simulink model "GaNModel_Nonsegmented"  (R2016a)
settings: Solver=VariableStepAuto  StartTime=0.0  StopTime=4e-5  MaxStep=0.01  RelTol=1e-3
values from neighbouring files (symbols this model uses):
  b1 = -8.43    [CapacitanceAnalytical.m]    (also in GanModel_Nonsegmented.m = 2.035; HalfBridge.m = 2.035; PoleZero.m = 3.944609415e-18)
  b2 = 42.2    [CapacitanceAnalytical.m]    (also in GanModel_Nonsegmented.m = 2.054; HalfBridge.m = 2.054; PoleZero.m = 7.00901047e-28)
  c1 = 30.26    [CapacitanceAnalytical.m]    (also in GanModel_Nonsegmented.m = 0.124; HalfBridge.m = 0.124; PoleZero.m = 5.00726198929e-08)
  c2 = 7.341    [CapacitanceAnalytical.m]    (also in GanModel_Nonsegmented.m = 0.153; HalfBridge.m = 0.153; PoleZero.m = 1.94274928479e-17)
  Cds = Coss - Crss    [CapacitanceAnalytical.m]    (also in GanModel_Nonsegmented.m = 1.65e-11; HalfBridge.m = 6.3e-11; HalfBridgeBottomConnectedLoad.m = 6.3e-11; HalfBridgeCapacitanceModelling.m = 6.3e-11)
  Cgd = Crss    [CapacitanceAnalytical.m]    (also in GanModel_Nonsegmented.m = 5e-13; HalfBridge.m = 2e-12; HalfBridgeBottomConnectedLoad.m = 2e-12; HalfBridgeCapacitanceModelling.m = 2e-12)
  Cgs = Ciss - Crss    [CapacitanceAnalytical.m]    (also in GanModel_Nonsegmented.m = 6.45e-11; HalfBridge.m = 2.58e-10; HalfBridgeBottomConnectedLoad.m = 2.58e-10; HalfBridgeCapacitanceModelling.m = 2.58e-10)
  d1 = 1.159    [GanModel_Nonsegmented.m]    (also in HalfBridge.m)
  e1 = -0.204    [GanModel_Nonsegmented.m]    (also in HalfBridge.m)
  fsw = 1e6    (= 1000000)    [ChannelAndDSTrajectories.m]    (also in GanModel_Nonsegmented.m = 100000; HalfBridge.m; HalfBridgeBottomConnectedLoad.m; HalfBridgeCapacitanceModelling.m)
  K1 = 0.283    [GanModel_Nonsegmented.m]    (also in HalfBridge.m)
  K2 = 7.114    [GanModel_Nonsegmented.m]    (also in HalfBridge.m)
  Ld = 10e-9    (= 1e-08)    [GanModel_Nonsegmented.m]    (also in HalfBridge.m = 7e-09; HalfBridgeBottomConnectedLoad.m = 7e-09; HalfBridgeCapacitanceModelling.m = 7e-10)
  m1 = 30.972    [GanModel_Nonsegmented.m]    (also in HalfBridge.m)
  n1 = -4.48    [GanModel_Nonsegmented.m]    (also in HalfBridge.m)
  PulseAmplitude = 5    [GanModel_Nonsegmented.m]    (also in HalfBridge.m; HalfBridgeBottomConnectedLoad.m; HalfBridgeCapacitanceModelling.m)
  Rd = 3.6*0.95*0.82*18.2*0.25/295    (= 0.0432543050847)    [AnalyticalModel.m]    (also in GanModel_Nonsegmented.m = 0.1; HalfBridge.m = 2.5e-05; HalfBridgeBottomConnectedLoad.m = 2.5e-05; HalfBridgeCapacitanceModelling.m = 2.5e-05)
  Rg = 1    [GanModel_Nonsegmented.m]    (also in HalfBridge.m; HalfBridgeBottomConnectedLoad.m = 1.5; HalfBridgeCapacitanceModelling.m = 1.5)
  Rs = 3.6*0.238*0.82/295    (= 0.00238161355932)    [AnalyticalModel.m]    (also in GanModel_Nonsegmented.m = 0.1; HalfBridge.m = 2.5e-05; HalfBridgeBottomConnectedLoad.m = 2.5e-05; HalfBridgeCapacitanceModelling.m = 2.5e-05)
  SampleTime = 1e-12    [GanModel_Nonsegmented.m]    (also in HalfBridge.m = 5e-13; HalfBridgeBottomConnectedLoad.m = 5e-13; HalfBridgeCapacitanceModelling.m = 5e-13)
  Vdc = 300    [GanModel_Nonsegmented.m]    (also in HalfBridge.m; HalfBridgeBottomConnectedLoad.m; HalfBridgeCapacitanceModelling.m)
libraries: powerlib x18
settings Model: Creator=ugurm  LastModifiedBy=ugurm
settings DebuggingCC: UnconnectedInputMsg=none  UnconnectedOutputMsg=none  UnconnectedLineMsg=none

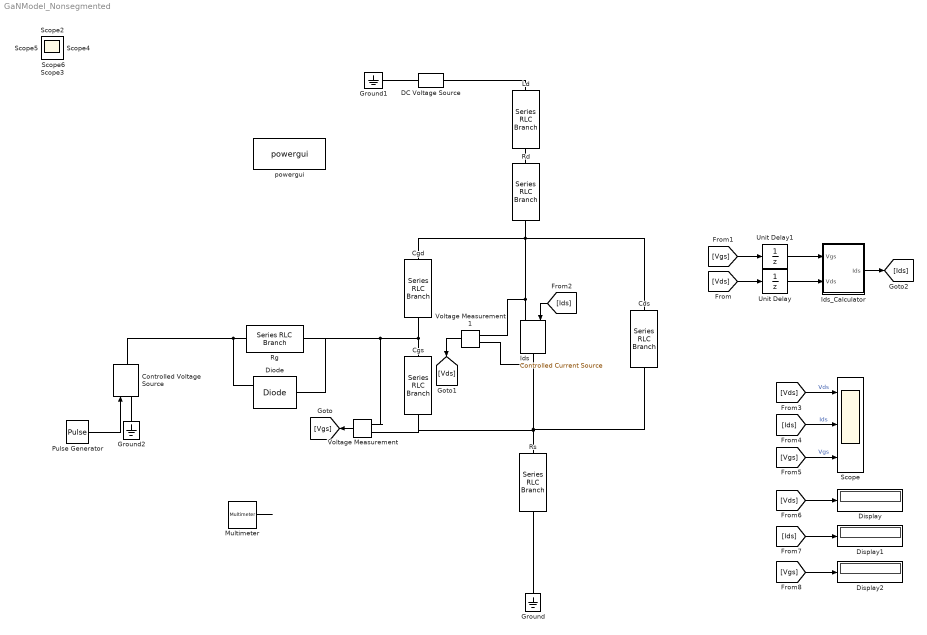
== system GaNModel_Nonsegmented ==
  Cds : powerlib/Elements/Series RLC Branch  LConnTagsString=__new0  RConnTagsString=__new0  BranchType=C  Resistance=1  Inductance=1e-3  SetiL0=off  InitialCurrent=0  Capacitance=Cds  Setx0=off  InitialVoltage=0  Measurements=None
  Cgd : powerlib/Elements/Series RLC Branch  LConnTagsString=__new0  RConnTagsString=__new0  BranchType=C  Resistance=1  Inductance=1e-3  SetiL0=off  InitialCurrent=0  Capacitance=Cgd  Setx0=off  InitialVoltage=0  Measurements=None
  Cgs : powerlib/Elements/Series RLC Branch  LConnTagsString=__new0  RConnTagsString=__new0  BranchType=C  Resistance=1  Inductance=1e-3  SetiL0=off  InitialCurrent=0  Capacitance=Cgs  Setx0=off  InitialVoltage=0  Measurements=None
  Controlled Voltage Source : powerlib/Electrical Sources/Controlled Voltage Source  Initialize=off  Source_Type=AC  Amplitude=0  Phase=0  Frequency=0  Measurements=Voltage
  DC Voltage Source : powerlib/Electrical Sources/DC Voltage Source  Amplitude=Vdc  Measurements=None
  Diode : powerlib/Power Electronics/Diode  Ron=0.001  Lon=0  Vf=0.8  IC=0  UseSnubber=off  Rs=500  Cs=250e-9  Measurements=on
  Display : Display
  Display1 : Display
  Display2 : Display
  Ground : powerlib/Elements/Ground  LConnTagsString=a
  Ground1 : powerlib/Elements/Ground  LConnTagsString=a
  Ground2 : powerlib/Elements/Ground  LConnTagsString=a
  Ids : powerlib/Electrical Sources/Controlled Current Source  Initialize=on  Source_Type=AC  Amplitude=0  Phase=0  Frequency=0  Measurements=None
  Ids_Calculator : Subsystem
  Ld : powerlib/Elements/Series RLC Branch  LConnTagsString=__new0  RConnTagsString=__new0  BranchType=L  Resistance=Rd  Inductance=Ld  SetiL0=off  InitialCurrent=0  Capacitance=1e-6  Setx0=off  InitialVoltage=0  Measurements=None
  Multimeter : powerlib/Measurements/Multimeter  PhasorSimulation=off  OutputType=Complex  sel=1  L=1  Gain=1  yselected={'Usrc: Controlled Voltage Source'};  PSBOutputType=1  PSBequivalent=0  AxesSetting=[0,0.1,-100,100]  Display=0  SavedBlockNames=-11
  Pulse Generator : DiscretePulseGenerator  PulseType=Time based  Amplitude=PulseAmplitude  Period=1/fsw  PulseWidth=50
  Rd : powerlib/Elements/Series RLC Branch  LConnTagsString=__new0  RConnTagsString=__new0  BranchType=R  Resistance=Rd  Inductance=1e-3  SetiL0=off  InitialCurrent=0  Capacitance=1e-6  Setx0=off  InitialVoltage=0  Measurements=None
  Rg : powerlib/Elements/Series RLC Branch  LConnTagsString=__new0  RConnTagsString=__new0  BranchType=R  Resistance=Rg  Inductance=1e-3  SetiL0=off  InitialCurrent=0  Capacitance=1e-6  Setx0=off  InitialVoltage=0  Measurements=None
  Rs : powerlib/Elements/Series RLC Branch  LConnTagsString=__new0  RConnTagsString=__new0  BranchType=R  Resistance=Rs  Inductance=1e-3  SetiL0=off  InitialCurrent=0  Capacitance=1e-6  Setx0=off  InitialVoltage=0  Measurements=None
  Scope : Scope  NumInputPorts=3
  Unit Delay : UnitDelay  SampleTime=-1
  Unit Delay1 : UnitDelay  SampleTime=-1
  Voltage Measurement : powerlib/Measurements/Voltage Measurement  PhasorSimulation=off  OutputType=Complex  PSBequivalent=0
  Voltage Measurement1 : powerlib/Measurements/Voltage Measurement  PhasorSimulation=off  OutputType=Complex  PSBequivalent=0
  powergui : powerlib/powergui  Priority=1  SimulationMode=Discrete  SolverType=Tustin/Backward Euler (TBE)  SampleTime=SampleTime  frequency=60  SPID=on  DisableSnubberDevices=on  DisableRonSwitches=off  DisableVfSwitches=off  SwTol=0  DisplayEquations=off  Interpol=on  ExternalGateDelay=on  methode=on  Ts=10  FunctionMessages=off  echomessages=off  HookPort=off  EnableUseOfTLC=off  x0status=blocks  frequencyindice=0  Pbase=100e6  ErrMax=1e-4  Iterations=50  UnitsV=kV  UnitsW=MW  buscounter=0  RestoreLinks=warning  ResistiveCurrentMeasurement=off  Frange=[0:2:500]  Ylog=off  Xlog=on  ShowGrid=off  save=off  variable=ZData  structure=0  ZoomFFT=off  StartTime=0.0  cycles=1  DisplayStyle=1  fundamental=60  FreqAxis=off  MaxFrequency=1000  frequencyindicesteady=1  RmsSteady=1  display=off
  Scope{1..6} (6 alike) : Scope
  wires:
  Voltage Measurement/1 -> [Vgs]
  Voltage Measurement1/1 -> [Vds]
  Ids_Calculator/1(Ids) -> [Ids]
  [Ids] -> Ids/1
  [Vds] -> Scope/1  "Vds"
  [Ids] -> Scope/2  "Ids"
  [Vgs] -> Scope/3  "Vgs"
  [Vgs] -> Unit Delay1/1
  [Vds] -> Unit Delay/1
  Unit Delay1/1 -> Ids_Calculator/1(Vgs)
  Unit Delay/1 -> Ids_Calculator/2(Vds)
  [Ids] -> Display1/1
  [Vds] -> Display/1
  [Vgs] -> Display2/1
  Pulse Generator/1 -> Controlled Voltage Source/1
  Multimeter/1 -> ?
  connections:
  Ids/LConn1 -- Voltage Measurement1/LConn1 -- Rd/RConn1 -- Cgd/LConn1 -- Cds/LConn1
  Ids/RConn1 -- Cds/RConn1 -- Cgs/RConn1 -- Voltage Measurement/LConn2 -- Rs/LConn1 -- Voltage Measurement1/LConn2
  Cgs/LConn1 -- Diode/LConn1 -- Rg/RConn1 -- Voltage Measurement/LConn1 -- Cgd/RConn1
  DC Voltage Source/RConn1 -- Ld/LConn1
  Ground1/LConn1 -- DC Voltage Source/LConn1
  Diode/RConn1 -- Rg/LConn1 -- Controlled Voltage Source/RConn1
  Controlled Voltage Source/LConn1 -- Ground2/LConn1
  Ld/RConn1 -- Rd/LConn1
  Ground/LConn1 -- Rs/RConn1

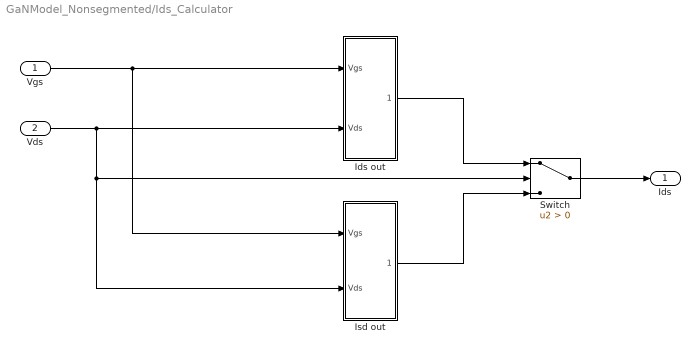
== system GaNModel_Nonsegmented/Ids_Calculator ==
  Vgs : Inport
  Vds : Inport  Port=2
  Ids out : Subsystem
  Isd out : Subsystem
  Switch : Switch  Criteria=u2 > Threshold
  Ids : Outport
  wires:
  Vgs/1 -> Isd out/1(Vgs), Ids out/1(Vgs)
  Vds/1 -> Switch/2, Isd out/2(Vds), Ids out/2(Vds)
  Ids out/1(Out1) -> Switch/1
  Isd out/1(Out1) -> Switch/3
  Switch/1 -> Ids/1

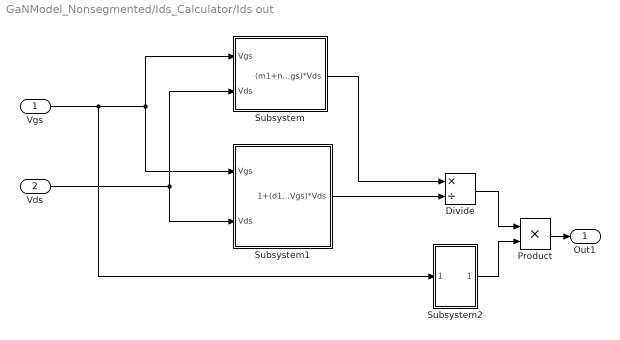
== system GaNModel_Nonsegmented/Ids_Calculator/Ids out ==
  Vgs : Inport
  Vds : Inport  Port=2
  Divide : Product  Inputs=*/
  Product : Product
  Subsystem : Subsystem
  Subsystem1 : Subsystem
  Subsystem2 : Subsystem
  Out1 : Outport
  wires:
  Subsystem1/1(1+(d1+e1*Vgs)*Vds) -> Divide/2
  Vds/1 -> Subsystem1/2(Vds), Subsystem/2(Vds)
  Vgs/1 -> Subsystem2/1(Vgs), Subsystem1/1(Vgs), Subsystem/1(Vgs)
  Subsystem/1((m1+n1*Vgs)*Vds) -> Divide/1
  Product/1 -> Out1/1
  Subsystem2/1(Out) -> Product/2
  Divide/1 -> Product/1

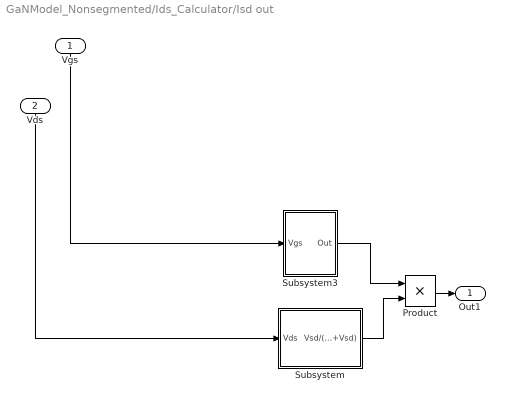
== system GaNModel_Nonsegmented/Ids_Calculator/Isd out ==
  Vgs : Inport
  Vds : Inport  Port=2
  Product : Product
  Subsystem : Subsystem
  Subsystem3 : Subsystem
  Out1 : Outport
  wires:
  Subsystem3/1(Out) -> Product/1
  Product/1 -> Out1/1
  Vgs/1 -> Subsystem3/1(Vgs)
  Vds/1 -> Subsystem/1(Vds)
  Subsystem/1(Vsd/(1+Vsd)) -> Product/2

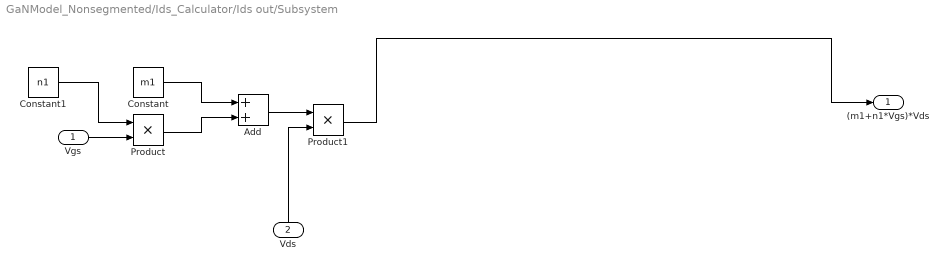
== system GaNModel_Nonsegmented/Ids_Calculator/Ids out/Subsystem ==
  Vgs : Inport
  Vds : Inport  Port=2
  Add : Sum
  Constant : Constant  Value=m1
  Constant1 : Constant  Value=n1
  Product : Product
  Product1 : Product
  (m1+n1*Vgs)*Vds : Outport
  wires:
  Constant1/1 -> Product/1
  Constant/1 -> Add/1
  Vds/1 -> Product1/2
  Vgs/1 -> Product/2
  Product/1 -> Add/2
  Product1/1 -> (m1+n1*Vgs)*Vds/1
  Add/1 -> Product1/1

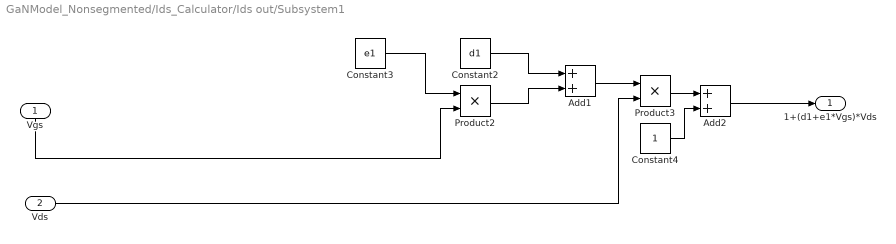
== system GaNModel_Nonsegmented/Ids_Calculator/Ids out/Subsystem1 ==
  Vgs : Inport
  Vds : Inport  Port=2
  Add1 : Sum
  Add2 : Sum
  Constant2 : Constant  Value=d1
  Constant3 : Constant  Value=e1
  Constant4 : Constant
  Product2 : Product
  Product3 : Product
  1+(d1+e1*Vgs)*Vds : Outport
  wires:
  Product2/1 -> Add1/2
  Add1/1 -> Product3/1
  Constant2/1 -> Add1/1
  Constant3/1 -> Product2/1
  Product3/1 -> Add2/1
  Vds/1 -> Product3/2
  Add2/1 -> 1+(d1+e1*Vgs)*Vds/1
  Vgs/1 -> Product2/2
  Constant4/1 -> Add2/2

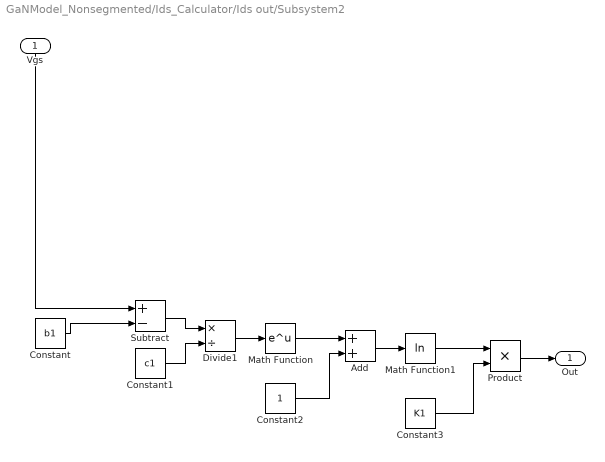
== system GaNModel_Nonsegmented/Ids_Calculator/Ids out/Subsystem2 ==
  Vgs : Inport
  Add : Sum
  Constant : Constant  Value=b1
  Constant1 : Constant  Value=c1
  Constant2 : Constant
  Constant3 : Constant  Value=K1
  Divide1 : Product  Inputs=*/
  Math Function : Math  SaturateOnIntegerOverflow=on
  Math Function1 : Math  Operator=log  RndMeth=Zero  SaturateOnIntegerOverflow=on
  Product : Product
  Subtract : Sum  Inputs=+-
  Out : Outport
  wires:
  Divide1/1 -> Math Function/1
  Constant1/1 -> Divide1/2
  Constant3/1 -> Product/2
  Product/1 -> Out/1
  Vgs/1 -> Subtract/1
  Constant/1 -> Subtract/2
  Math Function1/1 -> Product/1
  Math Function/1 -> Add/1
  Constant2/1 -> Add/2
  Subtract/1 -> Divide1/1
  Add/1 -> Math Function1/1

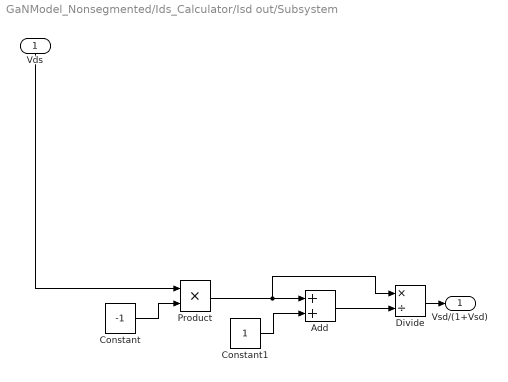
== system GaNModel_Nonsegmented/Ids_Calculator/Isd out/Subsystem ==
  Vds : Inport
  Add : Sum
  Constant : Constant  Value=-1
  Constant1 : Constant
  Divide : Product  Inputs=*/
  Product : Product
  Vsd/(1+Vsd) : Outport
  wires:
  Constant/1 -> Product/2
  Add/1 -> Divide/2
  Vds/1 -> Product/1
  Constant1/1 -> Add/2
  Divide/1 -> Vsd/(1+Vsd)/1
  Product/1 -> Divide/1, Add/1

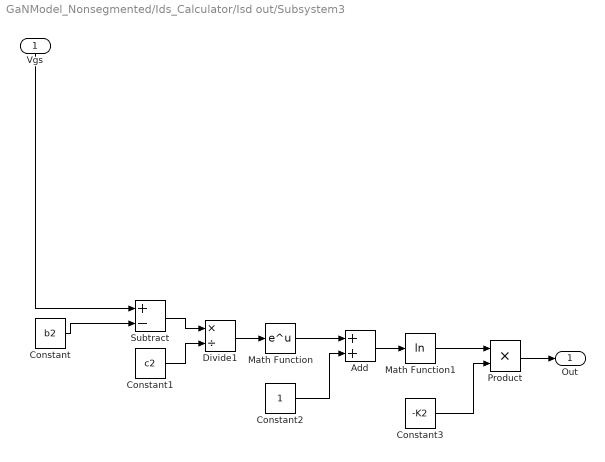
== system GaNModel_Nonsegmented/Ids_Calculator/Isd out/Subsystem3 ==
  Vgs : Inport
  Add : Sum
  Constant : Constant  Value=b2
  Constant1 : Constant  Value=c2
  Constant2 : Constant
  Constant3 : Constant  Value=-K2
  Divide1 : Product  Inputs=*/
  Math Function : Math  SaturateOnIntegerOverflow=on
  Math Function1 : Math  Operator=log  RndMeth=Zero  SaturateOnIntegerOverflow=on
  Product : Product
  Subtract : Sum  Inputs=+-
  Out : Outport
  wires:
  Add/1 -> Math Function1/1
  Subtract/1 -> Divide1/1
  Constant2/1 -> Add/2
  Math Function/1 -> Add/1
  Math Function1/1 -> Product/1
  Constant/1 -> Subtract/2
  Vgs/1 -> Subtract/1
  Product/1 -> Out/1
  Constant3/1 -> Product/2
  Constant1/1 -> Divide1/2
  Divide1/1 -> Math Function/1
